simulink model "Diskret_Regelkreis_P"  (R2021a)
settings: Solver=VariableStepAuto  StartTime=0.0  StopTime=0.4  RelTol=1e-3
model workspace (MAT data in the model file):
  K_p = 1
  T = 0.001
  T_1 = 0.01
  T_2 = 0.1
  n_soll = 1
  n_start = 0
  v = 4
libraries: Regler x4
settings Model: Creator=Manoli  LastModifiedBy=Manoli

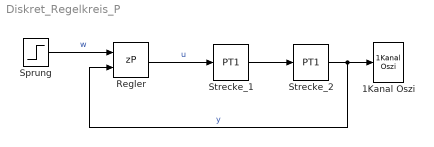
== system Diskret_Regelkreis_P ==
  1Kanal Oszi : Regler/1Kanal Oszi  TR=1  ymin=0  ymax=1  npts=inf  color='r-/b-/g-/m-'
  Regler : Regler/zP  kp=K_p  T=T
  Sprung : Step  Time=0.000001  Before=n_start  After=n_soll  SampleTime=0
  Strecke_1 : Regler/PT1  k=v  T1=T_1
  Strecke_2 : Regler/PT1  k=1  T1=T_2
  wires:
  Sprung/1 -> Regler/1  "w"
  Regler/1 -> Strecke_1/1  "u"
  Strecke_1/1 -> Strecke_2/1
  Strecke_2/1 -> Regler/2, 1Kanal Oszi/1  "y"
